simulink model "rotation_X_control_C2"  (R2016a)
settings: Solver=VariableStepAuto  StartTime=0.0  StopTime=10.0  RelTol=1e-3
undefined symbols (not defined in the file): g, m
settings Model: Creator=mgreiff  LastModifiedBy=mgreiff

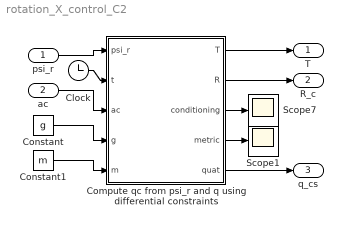
== system rotation_X_control_C2 ==
  psi_r : Inport  PortDimensions=1
  ac : Inport  Port=2  PortDimensions=3
  Clock : Clock
  Compute qc from psi_r and q using differential constraints : MATLAB Function  TreatAsAtomicUnit=on
  Constant : Constant  Value=g
  Constant1 : Constant  Value=m
  Scope1 : Scope
  Scope7 : Scope
  T : Outport  PortDimensions=1
  R_c : Outport  Port=2
  q_cs : Outport  Port=3  PortDimensions=4
  wires:
  psi_r/1 -> Compute qc from psi_r and q using differential constraints/1(psi_r)
  ac/1 -> Compute qc from psi_r and q using differential constraints/3(ac)
  Compute qc from psi_r and q using differential constraints/2(R) -> R_c/1
  Compute qc from psi_r and q using differential constraints/1(T) -> T/1
  Constant/1 -> Compute qc from psi_r and q using differential constraints/4(g)
  Constant1/1 -> Compute qc from psi_r and q using differential constraints/5(m)
  Compute qc from psi_r and q using differential constraints/5(quat) -> q_cs/1
  Compute qc from psi_r and q using differential constraints/3(conditioning) -> Scope7/1
  Compute qc from psi_r and q using differential constraints/4(metric) -> Scope1/1
  Clock/1 -> Compute qc from psi_r and q using differential constraints/2(t)

== matlab function rotation_X_control_C2/Compute qc from psi_r and q using differential constraints ==
  data: T output; R output; conditioning output; metric output; psi_r input; t input; ac input; g input; m input; quat output
function [T, R, conditioning, metric, quat]  = C2(psi_r, t, ac, g, m)
    % ~~~~~~~~~ Copyright (c) 2018 Marcus Greiff (see LICENCE.md) ~~~~~~~~~
    %
    % Computes a commanded attitude on SO(3) from a commanded acceleration
    % and the differential constraints of the UAV. This is done in a
    % singularity-free manner, where the lifting of the SO(3) rotation to
    % SO(4) is done using the eigenspace method.
    %
    %     [T, R, conditioning, metric, quat]  = C2(psi_r, t, ac, g, m)

    persistent zBprev;
    persistent tprev;
    persistent Rprev;
    persistent psiPrev;

    % Accelerations on the body
    atilde = ac + [0;0;g];
    T = m*norm(atilde);
        
    if isempty(zBprev) || isempty(tprev) || isempty(Rprev)|| isempty(psiPrev)
        zBprev = [0;0;1];
        psiPrev = psi_r;
        tprev = 0;
        Rprev = eye(3);
        R = eye(3);
    else

        % Compute the desired rotation
        zb = atilde./norm(atilde);
        v = cross(zBprev, zb);
        c = dot(zBprev, zb);
        dR = eye(3) + skew(v) + skew(v)*skew(v) ./ (1+c);
        dAng = (psi_r - psiPrev);

        R = dR*Rprev;
        R = R + R * skew([0;0;dAng]) + (1/2).*R*skew([0;0;dAng])*skew([0;0;dAng]);
        R = R./norm(R);
        Rprev = R;
        zBprev = zb;
        psiPrev = psi_r;
    end

    metric = 0;
    conditioning = 0;
    
    % Pre-allocate output
    quat = zeros(size(R,3), 4, 'like', R);

    % Calculate all elements of symmetric K matrix
    K11 = R(1,1,:) - R(2,2,:) - R(3,3,:);
    K12 = R(1,2,:) + R(2,1,:);
    K13 = R(1,3,:) + R(3,1,:);
    K14 = R(3,2,:) - R(2,3,:);
    K22 = R(2,2,:) - R(1,1,:) - R(3,3,:);
    K23 = R(2,3,:) + R(3,2,:);
    K24 = R(1,3,:) - R(3,1,:);
    K33 = R(3,3,:) - R(1,1,:) - R(2,2,:);
    K34 = R(2,1,:) - R(1,2,:);
    K44 = R(1,1,:) + R(2,2,:) + R(3,3,:);

    K = [...
        K11,    K12,    K13,    K14;
        K12,    K22,    K23,    K24;
        K13,    K23,    K33,    K34;
        K14,    K24,    K34,    K44] ./ 3;

    for i = 1:size(R,3)
        [eigVec,eigVal] = eig(K(:,:,i),'vector');
        [~,maxIdx] = max(real(eigVal));
        quat(i,:) = real([eigVec(4,maxIdx) eigVec(1,maxIdx) eigVec(2,maxIdx) eigVec(3,maxIdx)]);

        if quat(i,1) < 0
            quat(i,:) = -quat(i,:);
        end
    end
end


function S = skew(v)
    vx = v(1);
    vy = v(2);
    vz = v(3);
    S = [0 -vz vy; vz 0 -vx; -vy vx 0];
end
